simulink subsystem "Communication_Simulator"  (R2024a)
settings: Solver=VariableStepAuto  StartTime=0.0  StopTime=10.0  RelTol=1e-3
undefined symbols (not defined in the file): paramRFSatLink, QAM, rfSatSourceSamplesPerSymbol, rfSatSourceSampleTime
libraries: commrflib2 x24, dspsigops x12, commrfcorlib x8, commfilt2 x8, commdigbbndam3 x8, dspsolvers x8, simulink x8, commrandsrc3 x4, commsink2 x4, commdemoslib x4, impairlib x4, commsync2 x4
(part 2 of 3)

== system Communication_Simulator/TT&C Communication/Ground Segment/BER Calculation ==
  note: BER Results (with reset)
  note: Bits
  note: Errors
  note: BER
  BER Measurements : Display
  Constant : Constant  Value=paramRFSatLink.resetBER  SampleTime=rfSatSourceSampleTime * rfSatSourceSamplesPerSymbol
  Error Rate Calculation : commsink2/Error Rate Calculation  N=24  st_delay=0  cp_mode=Entire frame  subframe=[]  PMode=Port  WsName=ErrorVec  RsMode2=on  stop=off  numErr=200  maxBits=1e6
  Selector : Selector  InputPortWidth=3  IndexOptions=Index vector (dialog)  Indices=[1]  OutputSizes=1
  BER : Outport  VectorParamsAs1DForOutWhenUnconnected=off
  wires:
  [RF_downlink_Tx] -> Error Rate Calculation/1
  Selector/1 -> BER/1
  Constant/1 -> Error Rate Calculation/3
  Error Rate Calculation/1 -> BER Measurements/1, Selector/1
  [RF_downlink_Rx] -> Error Rate Calculation/2

== system Communication_Simulator/TT&C Communication/Ground Segment/BER Calculation1 ==
  note: BER Results (with reset)
  note: Bits
  note: Errors
  note: BER
  BER Measurements : Display
  Constant : Constant  Value=paramRFSatLink.resetBER  SampleTime=rfSatSourceSampleTime * rfSatSourceSamplesPerSymbol
  Error Rate Calculation : commsink2/Error Rate Calculation  N=24  st_delay=0  cp_mode=Entire frame  subframe=[]  PMode=Port  WsName=ErrorVec  RsMode2=on  stop=off  numErr=200  maxBits=1e6
  Selector : Selector  InputPortWidth=3  IndexOptions=Index vector (dialog)  Indices=[1]  OutputSizes=1
  BER : Outport  VectorParamsAs1DForOutWhenUnconnected=off
  wires:
  [RF_uplink_Tx] -> Error Rate Calculation/1
  Selector/1 -> BER/1
  Constant/1 -> Error Rate Calculation/3
  Error Rate Calculation/1 -> BER Measurements/1, Selector/1
  [RF_uplink_Rx] -> Error Rate Calculation/2

== system Communication_Simulator/TT&C Communication/Ground Segment/Close Plots ==

== system Communication_Simulator/TT&C Communication/Ground Segment/Close Plots1 ==

== system Communication_Simulator/TT&C Communication/Ground Segment/Close Plots10 ==

== system Communication_Simulator/TT&C Communication/Ground Segment/Close Plots11 ==

== system Communication_Simulator/TT&C Communication/Ground Segment/Close Plots12 ==

== system Communication_Simulator/TT&C Communication/Ground Segment/Close Plots13 ==

== system Communication_Simulator/TT&C Communication/Ground Segment/Close Plots14 ==

== system Communication_Simulator/TT&C Communication/Ground Segment/Close Plots15 ==

== system Communication_Simulator/TT&C Communication/Ground Segment/Close Plots2 ==

== system Communication_Simulator/TT&C Communication/Ground Segment/Close Plots3 ==

== system Communication_Simulator/TT&C Communication/Ground Segment/Close Plots4 ==

== system Communication_Simulator/TT&C Communication/Ground Segment/Close Plots5 ==

== system Communication_Simulator/TT&C Communication/Ground Segment/Close Plots6 ==

== system Communication_Simulator/TT&C Communication/Ground Segment/Close Plots7 ==

== system Communication_Simulator/TT&C Communication/Ground Segment/Close Plots8 ==

== system Communication_Simulator/TT&C Communication/Ground Segment/Close Plots9 ==

== system Communication_Simulator/TT&C Communication/Ground Segment/Downlink ==
  note: Downlink Path
  note: Satellite Downlink Transmitter
  note: Transmitter
  Telemetry : Inport
  Doppler Error : commrflib2/Phase// Frequency Offset  phaseOffset=0  freqPort=off  freqOffset=paramRFSatLink.DoppOffset
  Downlink Path : commrflib2/Free Space Path Loss  mode=Distance and Frequency  dB=180  d=paramRFSatLink.Altitude  fc=paramRFSatLink.Frequency
  Nonlinearity : Subsystem
      mask Display: disp('HPA\n Nonlinearity\n with Optional\n Digital\nPredistortion')
  Raised Cosine Transmit Filter : commfilt2/Raised Cosine Transmit Filter  filtType=Square root  R=0.3  filtSpan=paramRFSatLink.FilterSpan  N=paramRFSatLink.SamplesPerSymbol  filterGain=sqrt(paramRFSatLink.SamplesPerSymbol)  InputProcessing=Columns as channels (frame based)  RateOptions=Enforce single-rate processing  framing=Mute  checkCoeff=off  variableName=rcTxFilt  checkGain=Normalized  sampMode=Mute  saveAsFlag=0  currentFiltSpan=2*((2*(3))/2)  D=(2*(3))/2  launchFVT=off  roundingMode=Floor  overflowMode=off  coeffDataTypeStr=Inherit: Same word length as input  coeffMin=[]  coeffMax=[]  coeffLastDataTypeStr=Inherit: Same word length as input  outputDataTypeStr=Inherit: Same as accumulator  outputMin=[]  outputMax=[]  outputLastDataTypeStr=Inherit: Same as accumulator
  Rectangular QAM Modulator Baseband : commdigbbndam3/Rectangular QAM Modulator Baseband  M=16  InType=Bit  Enc=Gray  Mapping=[0:15]  PowType=Average Power  MinDist=2  AvgPow=2  PeakPow=1  Ph=0  outDtype=double  outWordLen=16  outUDDataType=sfix(16)  outFracLenMode=Best precision  outFracLen=15  outDataTypeStr=double  outLastDataTypeStr=double
  Tx Dish Antenna Gain : Gain  Gain=paramRFSatLink.TXAntGain_Downlink  SaturateOnIntegerOverflow=on  OutDataTypeStr=Inherit: Same as input  ParamDataTypeStr=Inherit: Same as input
  gs_rx_sig : Outport
  tag scope: RF_downlink_Tx=global, Tx_downlink_Ampl=global, Tx_downlink_RRC=global
  wires:
  Tx Dish Antenna Gain/1 -> Downlink Path/1
  Downlink Path/1 -> Doppler Error/1
  Doppler Error/1 -> gs_rx_sig/1
  Telemetry/1 -> [RF_downlink_Tx], Rectangular QAM Modulator Baseband/1
  Nonlinearity/1(Out2) -> Tx Dish Antenna Gain/1, [Tx_downlink_Ampl]
  Rectangular QAM Modulator Baseband/1 -> Raised Cosine Transmit Filter/1
  Raised Cosine Transmit Filter/1 -> Nonlinearity/1(In), [Tx_downlink_RRC]

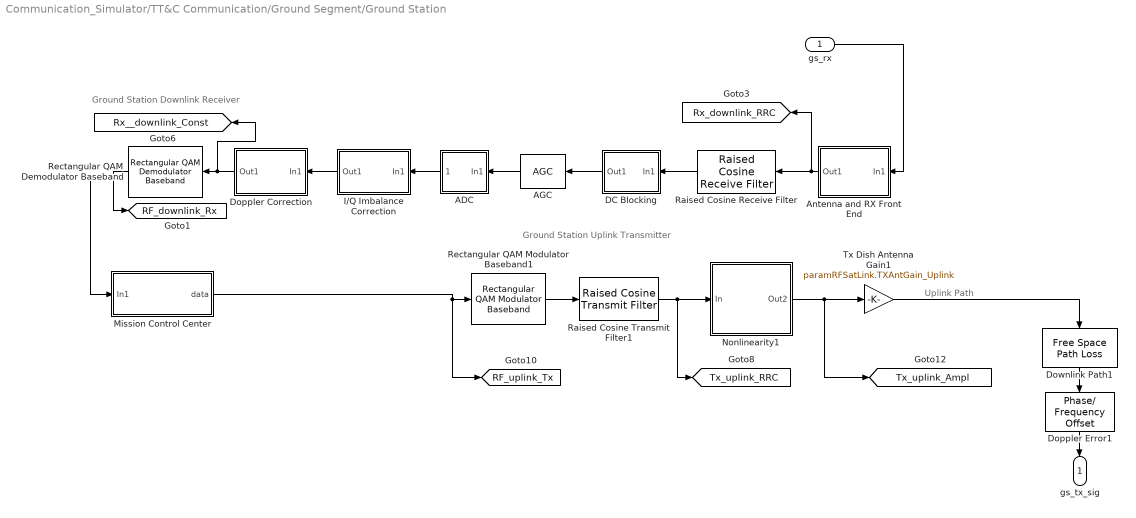
== system Communication_Simulator/TT&C Communication/Ground Segment/Ground Station ==
  note: Uplink Path
  note: Ground Station Uplink Transmitter
  note: Ground Station Downlink Receiver
  gs_rx : Inport
  ADC : Subsystem
      mask Display: disp('Bipolar\nADC')
  AGC : commrfcorlib/AGC  LegacyMode=off  DetectorMethod=Rectifier  LoopMethod=Linear  UpdatePeriod=100  StepSize=0.1  AdaptationStepSize=0.01  DesiredOutputPower=1  AveragingLength=256  MaximumGain=30  MaxPowerGain=400  GainOutputPort=off  InputPowerOutputPort=off  SimulateUsing=Code generation
  Antenna and RX Front End : Subsystem
      mask Display: disp('Antenna\nand\nRX Front End')
  DC Blocking : Subsystem
      mask Display: disp('DC\nBlocking')
  Doppler Correction : Subsystem
      mask Display: disp('Doppler\nCorrection')
  Doppler Error1 : commrflib2/Phase// Frequency Offset  phaseOffset=0  freqPort=off  freqOffset=paramRFSatLink.DoppOffset
  Downlink Path1 : commrflib2/Free Space Path Loss  mode=Distance and Frequency  dB=180  d=paramRFSatLink.Altitude  fc=paramRFSatLink.Frequency
  I/Q Imbalance Correction : Subsystem
      mask Display: disp('I/Q Imbalance\nCorrection')
  Mission Control Center : Subsystem
  Nonlinearity1 : Subsystem
      mask Display: disp('HPA\n Nonlinearity\n with Optional\n Digital\nPredistortion')
  Raised Cosine Receive Filter : commfilt2/Raised Cosine Receive Filter  filtType=Square root  R=0.3  filtSpan=paramRFSatLink.FilterSpan  N=paramRFSatLink.SamplesPerSymbol  downFactor=paramRFSatLink.SamplesPerSymbol  downOffset=0  filterGain=1/sqrt(paramRFSatLink.SamplesPerSymbol)  InputProcessing=Columns as channels (frame based)  RateOptions=Enforce single-rate processing  framing=Mute  checkCoeff=off  variableName=rcRxFilt  currentFiltSpan=2*((2*(3))/2)  D=(2*(3))/2  inputOffset=0  sampMode=Mute  saveAsFlag=0  rateMode=Downsampling  checkGain=Normalized  launchFVT=off  roundingMode=Floor  overflowMode=off  coeffDataTypeStr=Inherit: Same word length as input  coeffMin=[]  coeffMax=[]  coeffLastDataTypeStr=Inherit: Same word length as input  accumDataTypeStr=Inherit: Same as product output  accumLastDataTypeStr=Inherit: Same as product output  outputDataTypeStr=Inherit: Same as accumulator  outputMin=[]  outputMax=[]  outputLastDataTypeStr=Inherit: Same as accumulator
  Raised Cosine Transmit Filter1 : commfilt2/Raised Cosine Transmit Filter  filtType=Square root  R=0.3  filtSpan=paramRFSatLink.FilterSpan  N=paramRFSatLink.SamplesPerSymbol  filterGain=sqrt(paramRFSatLink.SamplesPerSymbol)  InputProcessing=Columns as channels (frame based)  RateOptions=Enforce single-rate processing  framing=Mute  checkCoeff=off  variableName=rcTxFilt1  checkGain=Normalized  sampMode=Mute  saveAsFlag=0  currentFiltSpan=2*((2*(3))/2)  D=(2*(3))/2  launchFVT=off  roundingMode=Floor  overflowMode=off  coeffDataTypeStr=Inherit: Same word length as input  coeffMin=[]  coeffMax=[]  coeffLastDataTypeStr=Inherit: Same word length as input  outputDataTypeStr=Inherit: Same as accumulator  outputMin=[]  outputMax=[]  outputLastDataTypeStr=Inherit: Same as accumulator
  Rectangular QAM Demodulator Baseband : commdigbbndam3/Rectangular QAM Demodulator Baseband  M=16  OutType=Bit  DecType=Hard decision  VarSource=Dialog  Variance=1  Dec=Gray  Mapping=[0:15]  PowType=Average Power  MinDist=2  AvgPow=2  PeakPow=1  Ph=0  outDtype1=double  outDtype2=double  derotateFactorWordLen=16  derotateFactorDataTypeStr=Inherit: Same word length as input  derotateFactorLastDataTypeStr=Inherit: Same word length as input  denormFactorWordLen=16  denormFactorDataTypeStr=Inherit: Same word length as input  denormFactorLastDataTypeStr=Inherit: Same word length as input  prodOutWordLen=32  prodOutOverflowMode=Wrap  prodOutRoundingMode=Floor  prodOutOvFlMode=off  prodOutOvFlModeLastStrValue=off  sumWordLen=32
  Rectangular QAM Modulator Baseband1 : commdigbbndam3/Rectangular QAM Modulator Baseband  M=16  InType=Bit  Enc=Gray  Mapping=[0:15]  PowType=Average Power  MinDist=2  AvgPow=1  PeakPow=1  Ph=0  outDtype=double  outWordLen=16  outUDDataType=sfix(16)  outFracLenMode=Best precision  outFracLen=15  outDataTypeStr=double  outLastDataTypeStr=double
  Tx Dish Antenna Gain1 : Gain  Gain=paramRFSatLink.TXAntGain_Uplink  SaturateOnIntegerOverflow=on  OutDataTypeStr=Inherit: Same as input  ParamDataTypeStr=Inherit: Same as input
  gs_tx_sig : Outport
  tag scope: RF_downlink_Rx=global, RF_uplink_Tx=global, Rx__downlink_Const=global, Rx_downlink_RRC=global, Tx_uplink_Ampl=global, Tx_uplink_RRC=global
  wires:
  Doppler Error1/1 -> gs_tx_sig/1
  Downlink Path1/1 -> Doppler Error1/1
  Tx Dish Antenna Gain1/1 -> Downlink Path1/1
  Rectangular QAM Modulator Baseband1/1 -> Raised Cosine Transmit Filter1/1
  Nonlinearity1/1(Out2) -> Tx Dish Antenna Gain1/1, [Tx_uplink_Ampl]
  Raised Cosine Transmit Filter1/1 -> Nonlinearity1/1(In), [Tx_uplink_RRC]
  Mission Control Center/1(data) -> [RF_uplink_Tx], Rectangular QAM Modulator Baseband1/1
  I/Q Imbalance Correction/1(Out1) -> Doppler Correction/1(In1)
  Antenna and RX Front End/1(Out1) -> [Rx_downlink_RRC], Raised Cosine Receive Filter/1
  DC Blocking/1(Out1) -> AGC/1
  ADC/1(Out2) -> I/Q Imbalance Correction/1(In1)
  Doppler Correction/1(Out1) -> Rectangular QAM Demodulator Baseband/1, [Rx__downlink_Const]
  AGC/1 -> ADC/1(In1)
  gs_rx/1 -> Antenna and RX Front End/1(In1)
  Raised Cosine Receive Filter/1 -> DC Blocking/1(In1)
  Rectangular QAM Demodulator Baseband/1 -> [RF_downlink_Rx], Mission Control Center/1(In1)

== system Communication_Simulator/TT&C Communication/Ground Segment/HPA ==
  HPA Input : Inport
  HPA Output : Inport  Port=2
  Matrix Concatenate : Concatenate  Mode=Multidimensional array  ConcatenateDimension=2
  RRC signal before and after HPA : ConstellationDiagram  WindowPosition=[508.333333333333 347.666666666667 282 242.666666666667]  SamplesPerSymbol=8  SymbolsToDisplaySource=Property  SymbolsToDisplay=1000  ReferenceConstellation=16-QAM  Title=RRC Signal Before and After HPA  XLimits=[-3.9233 3.9259]  YLimits=[-3.9233 3.9259]  ShowLegend=on  ShowReferenceConstellation=off  ColorFading=on  DefaultConfigurationName=comm.scopes.ConstellationDiagramBlockCfg
      settings: OpenAtSimulationStart=off
  wires:
  Matrix Concatenate/1 -> RRC signal before and after HPA/1
  HPA Output/1 -> Matrix Concatenate/2
  HPA Input/1 -> Matrix Concatenate/1

== system Communication_Simulator/TT&C Communication/Ground Segment/HPA1 ==
  HPA Input : Inport
  HPA Output : Inport  Port=2
  Matrix Concatenate : Concatenate  Mode=Multidimensional array  ConcatenateDimension=2
  RRC signal before and after HPA : ConstellationDiagram  WindowPosition=[508.333333333333 347.666666666667 282 242.666666666667]  SamplesPerSymbol=8  SymbolsToDisplaySource=Property  SymbolsToDisplay=1000  ReferenceConstellation=16-QAM  Title=RRC Signal Before and After HPA  XLimits=[-3.9233 3.9259]  YLimits=[-3.9233 3.9259]  ShowLegend=on  ShowReferenceConstellation=off  ColorFading=on  DefaultConfigurationName=comm.scopes.ConstellationDiagramBlockCfg
      settings: OpenAtSimulationStart=off
  wires:
  Matrix Concatenate/1 -> RRC signal before and after HPA/1
  HPA Output/1 -> Matrix Concatenate/2
  HPA Input/1 -> Matrix Concatenate/1

== system Communication_Simulator/TT&C Communication/Ground Segment/Input&Output of HPA ==
  In1 : Inport
  In2 : Inport  Port=2
  Add : Sum  Inputs=-+
  Complex to Magnitude-Angle : ComplexToMagnitudeAngle
  Complex to Magnitude-Angle1 : ComplexToMagnitudeAngle
  HPA AM to AM : ConstellationDiagram  Tag=ScatterPlot  WindowPosition=[1104 604 253 220]  SymbolsToDisplaySource=Property  SymbolsToDisplay=1000  Title=HPA AM to AM  XLimits=[-1.4713 6.1709]  YLimits=[-1.4713 6.1709]  XLabel=Input Amplitude  YLabel=Output Amplitude  ShowReferenceConstellation=off  ColorFading=on  DefaultConfigurationName=comm.scopes.ConstellationDiagramBlockCfg
      settings: OpenAtSimulationStart=off
  HPA AM to PM : ConstellationDiagram  Tag=ScatterPlot  WindowPosition=[842 605 253 220]  SymbolsToDisplaySource=Property  SymbolsToDisplay=1000  Title=HPA AM to PM  XLimits=[-1.0435 2.3201]  YLimits=[-1.0435 2.3201]  XLabel=Input Amplitude  YLabel=Phase Difference (rad)  ShowReferenceConstellation=off  ColorFading=on  DefaultConfigurationName=comm.scopes.ConstellationDiagramBlockCfg
      settings: OpenAtSimulationStart=off
  Real-Imag to Complex : RealImagToComplex
  Real-Imag to Complex1 : RealImagToComplex
  Unwrap : dspsigops/Unwrap  tol=pi  InputProcessing=Columns as channels (frame based)  running=on
  wires:
  Complex to Magnitude-Angle/2 -> Add/1
  Complex to Magnitude-Angle/1 -> Real-Imag to Complex/1, Real-Imag to Complex1/1
  Complex to Magnitude-Angle1/2 -> Add/2
  Unwrap/1 -> Real-Imag to Complex1/2
  Real-Imag to Complex1/1 -> HPA AM to PM/1
  In2/1 -> Complex to Magnitude-Angle1/1
  In1/1 -> Complex to Magnitude-Angle/1
  Add/1 -> Unwrap/1
  Complex to Magnitude-Angle1/1 -> Real-Imag to Complex/2
  Real-Imag to Complex/1 -> HPA AM to AM/1

== system Communication_Simulator/TT&C Communication/Ground Segment/Input&Output of HPA1 ==
  In1 : Inport
  In2 : Inport  Port=2
  Add : Sum  Inputs=-+
  Complex to Magnitude-Angle : ComplexToMagnitudeAngle
  Complex to Magnitude-Angle1 : ComplexToMagnitudeAngle
  HPA AM to AM : ConstellationDiagram  Tag=ScatterPlot  WindowPosition=[1104 604 253 220]  SymbolsToDisplaySource=Property  SymbolsToDisplay=1000  Title=HPA AM to AM  XLimits=[-1.4713 6.1709]  YLimits=[-1.4713 6.1709]  XLabel=Input Amplitude  YLabel=Output Amplitude  ShowReferenceConstellation=off  ColorFading=on  DefaultConfigurationName=comm.scopes.ConstellationDiagramBlockCfg
      settings: OpenAtSimulationStart=off
  HPA AM to PM : ConstellationDiagram  Tag=ScatterPlot  WindowPosition=[842 605 253 220]  SymbolsToDisplaySource=Property  SymbolsToDisplay=1000  Title=HPA AM to PM  XLimits=[-1.0435 2.3201]  YLimits=[-1.0435 2.3201]  XLabel=Input Amplitude  YLabel=Phase Difference (rad)  ShowReferenceConstellation=off  ColorFading=on  DefaultConfigurationName=comm.scopes.ConstellationDiagramBlockCfg
      settings: OpenAtSimulationStart=off
  Real-Imag to Complex : RealImagToComplex
  Real-Imag to Complex1 : RealImagToComplex
  Unwrap : dspsigops/Unwrap  tol=pi  InputProcessing=Columns as channels (frame based)  running=on
  wires:
  Complex to Magnitude-Angle/2 -> Add/1
  Complex to Magnitude-Angle/1 -> Real-Imag to Complex/1, Real-Imag to Complex1/1
  Complex to Magnitude-Angle1/2 -> Add/2
  Unwrap/1 -> Real-Imag to Complex1/2
  Real-Imag to Complex1/1 -> HPA AM to PM/1
  In2/1 -> Complex to Magnitude-Angle1/1
  In1/1 -> Complex to Magnitude-Angle/1
  Add/1 -> Unwrap/1
  Complex to Magnitude-Angle1/1 -> Real-Imag to Complex/2
  Real-Imag to Complex/1 -> HPA AM to AM/1

== system Communication_Simulator/TT&C Communication/Ground Segment/Power Spectrum ==
  In1 : Inport
  In2 : Inport  Port=2
  Matrix Concatenation : Concatenate  Mode=Multidimensional array  ConcatenateDimension=2
  Tx and Rx Spectrum : SpectrumAnalyzer  WindowPosition=[1.000000,41.000000,1020.000000,357.000000,]  ScopeFrameLocation=window  Method=Welch  SampleRate=200000  Span=200000  StartFrequency=-100000  StopFrequency=100000  AveragingMethod=Running  YLimits=[-132.25324983,35.45221687]  ShowLegend=on  ChannelNames="[\"Tramsitted \",\"Received\"]"  SelectedToolstripTab=spectrumAnalyzerToolstrip.spectrumTab  AllowFFTLengthLessThanSamplesPerUpdate=on  DefaultConfigurationName=spbscopes.SpectrumAnalyzerBlockCfg  IsFrequencyInputMode=0  FrequencyVectorPort=0  FrequencyVectorFromPort=0  FrequencyInputRBWPort=0  FrequencyInputRBWFromPort=0
  wires:
  Matrix Concatenation/1 -> Tx and Rx Spectrum/1
  In2/1 -> Matrix Concatenation/2
  In1/1 -> Matrix Concatenation/1

== system Communication_Simulator/TT&C Communication/Ground Segment/Power Spectrum1 ==
  In1 : Inport
  In2 : Inport  Port=2
  Matrix Concatenation : Concatenate  Mode=Multidimensional array  ConcatenateDimension=2
  Tx and Rx Spectrum : SpectrumAnalyzer  WindowPosition=[25 331 480 288]  Method=Welch  SampleRate=200000  Span=200000  StartFrequency=-100000  StopFrequency=100000  AveragingMethod=Running  YLimits=[-90.208205220815884218,27.456041881558888917]  ShowLegend=on  ChannelNames="[\"Tramsitted \",\"Received\"]"  AllowFFTLengthLessThanSamplesPerUpdate=on  DefaultConfigurationName=spbscopes.SpectrumAnalyzerBlockCfg  IsFrequencyInputMode=0  FrequencyVectorPort=0  FrequencyVectorFromPort=0  FrequencyInputRBWPort=0  FrequencyInputRBWFromPort=0
      settings: OpenAtSimulationStart=off
  wires:
  Matrix Concatenation/1 -> Tx and Rx Spectrum/1
  In2/1 -> Matrix Concatenation/2
  In1/1 -> Matrix Concatenation/1

== system Communication_Simulator/TT&C Communication/Ground Segment/Subsystem ==

== system Communication_Simulator/TT&C Communication/Ground Segment/Subsystem1 ==

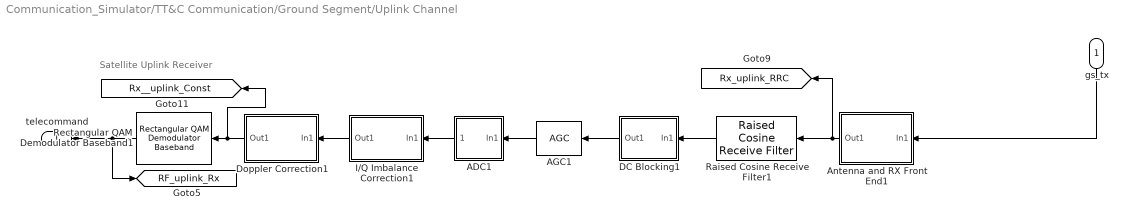
== system Communication_Simulator/TT&C Communication/Ground Segment/Uplink Channel ==
  note: Satellite Uplink Receiver
  gs_tx : Inport
  ADC1 : Subsystem
      mask Display: disp('Bipolar\nADC')
  AGC1 : commrfcorlib/AGC  LegacyMode=off  DetectorMethod=Rectifier  LoopMethod=Linear  UpdatePeriod=100  StepSize=0.1  AdaptationStepSize=0.01  DesiredOutputPower=1  AveragingLength=256  MaximumGain=30  MaxPowerGain=400  GainOutputPort=off  InputPowerOutputPort=off  SimulateUsing=Code generation
  Antenna and RX Front End1 : Subsystem
      mask Display: disp('Antenna\nand\nRX Front End')
  DC Blocking1 : Subsystem
      mask Display: disp('DC\nBlocking')
  Doppler Correction1 : Subsystem
      mask Display: disp('Doppler\nCorrection')
  I/Q Imbalance Correction1 : Subsystem
      mask Display: disp('I/Q Imbalance\nCorrection')
  Raised Cosine Receive Filter1 : commfilt2/Raised Cosine Receive Filter  filtType=Square root  R=0.3  filtSpan=paramRFSatLink.FilterSpan  N=paramRFSatLink.SamplesPerSymbol  downFactor=paramRFSatLink.SamplesPerSymbol  downOffset=0  filterGain=1/sqrt(paramRFSatLink.SamplesPerSymbol)  InputProcessing=Columns as channels (frame based)  RateOptions=Enforce single-rate processing  framing=Mute  checkCoeff=off  variableName=rcRxFilt1  currentFiltSpan=2*((2*(3))/2)  D=(2*(3))/2  inputOffset=0  sampMode=Mute  saveAsFlag=0  rateMode=Downsampling  checkGain=Normalized  launchFVT=off  roundingMode=Floor  overflowMode=off  coeffDataTypeStr=Inherit: Same word length as input  coeffMin=[]  coeffMax=[]  coeffLastDataTypeStr=Inherit: Same word length as input  accumDataTypeStr=Inherit: Same as product output  accumLastDataTypeStr=Inherit: Same as product output  outputDataTypeStr=Inherit: Same as accumulator  outputMin=[]  outputMax=[]  outputLastDataTypeStr=Inherit: Same as accumulator
  Rectangular QAM Demodulator Baseband1 : commdigbbndam3/Rectangular QAM Demodulator Baseband  M=16  OutType=Bit  DecType=Hard decision  VarSource=Dialog  Variance=1  Dec=Gray  Mapping=[0:15]  PowType=Average Power  MinDist=2  AvgPow=1  PeakPow=1  Ph=0  outDtype1=double  outDtype2=double  derotateFactorWordLen=16  derotateFactorDataTypeStr=Inherit: Same word length as input  derotateFactorLastDataTypeStr=Inherit: Same word length as input  denormFactorWordLen=16  denormFactorDataTypeStr=Inherit: Same word length as input  denormFactorLastDataTypeStr=Inherit: Same word length as input  prodOutWordLen=32  prodOutOverflowMode=Wrap  prodOutRoundingMode=Floor  prodOutOvFlMode=off  prodOutOvFlModeLastStrValue=off  sumWordLen=32
  telecommand : Outport
  tag scope: RF_uplink_Rx=global, Rx__uplink_Const=global, Rx_uplink_RRC=global
  wires:
  gs_tx/1 -> Antenna and RX Front End1/1(In1)
  I/Q Imbalance Correction1/1(Out1) -> Doppler Correction1/1(In1)
  Rectangular QAM Demodulator Baseband1/1 -> [RF_uplink_Rx], telecommand/1
  AGC1/1 -> ADC1/1(In1)
  Raised Cosine Receive Filter1/1 -> DC Blocking1/1(In1)
  ADC1/1(Out2) -> I/Q Imbalance Correction1/1(In1)
  Antenna and RX Front End1/1(Out1) -> [Rx_uplink_RRC], Raised Cosine Receive Filter1/1
  Doppler Correction1/1(Out1) -> Rectangular QAM Demodulator Baseband1/1, [Rx__uplink_Const]
  DC Blocking1/1(Out1) -> AGC1/1

== system Communication_Simulator/TT&C Communication/Ground Segment/background11 ==

== system Communication_Simulator/TT&C Communication/Ground Segment/background12 ==

== system Communication_Simulator/TT&C Communication/Ground Segment/background13 ==

== system Communication_Simulator/TT&C Communication/Ground Segment/background14 ==

== system Communication_Simulator/TT&C Communication/Ground Segment/background4 ==

== system Communication_Simulator/TT&C Communication/Ground Segment/background5 ==

== system Communication_Simulator/TT&C Communication/Ground Segment/background6 ==

== system Communication_Simulator/TT&C Communication/Ground Segment/background7 ==

== system Communication_Simulator/ISL Payload (SPARCS-B) /ISL/ISL Receiver/ADC1 ==
  In1 : Inport
  ADC Control : Constant  Value=paramRFSatLink.ADC  SampleTime=rfSatSourceSampleTime * rfSatSourceSamplesPerSymbol
  Bipolar ADC : commdemoslib/Bipolar ADC  FS_V=paramRFSatLink.ADC_VFS  N=paramRFSatLink.ADC_NumBits
  Switch : Switch  Criteria=u2 ~= 0  SaturateOnIntegerOverflow=off  InputSameDT=off
  Out2 : Outport  VectorParamsAs1DForOutWhenUnconnected=off
  wires:
  Switch/1 -> Out2/1
  In1/1 -> Switch/3, Bipolar ADC/1
  ADC Control/1 -> Switch/2
  Bipolar ADC/1 -> Switch/1

== system Communication_Simulator/ISL Payload (SPARCS-B) /ISL/ISL Receiver/Antenna and RX Front End1 ==
  In1 : Inport
  I/Q Imbalance : commrflib2/I//Q Imbalance  ampImbal=paramRFSatLink.IQImbal(1)  phsImbal=paramRFSatLink.IQImbal(2)  Idc=paramRFSatLink.IQImbal(3)  Qdc=paramRFSatLink.IQImbal(4)
  LNA : Gain  Gain=1e6
  Phase Noise : impairlib/Phase Noise  Level=rfSatPhaseNoise  FrequencyOffset=100  SampleRate=2e5  RandomStream=mt19937ar with seed  Seed=2137  SimulateUsing=Interpreted execution
  Rx Dish Antenna Gain : Gain  Gain=paramRFSatLink.RXAntGain_ISL  SaturateOnIntegerOverflow=on  OutDataTypeStr=Inherit: Same as input  ParamDataTypeStr=Inherit: Same as input
  Satellite Receiver System Temp : commrflib2/Receiver Thermal Noise  LegacyMode=on  NoiseMethod=Noise temperature  NoiseTemperature=paramRFSatLink.RXTemp  NoiseFigure=20  NoiseFactor=2  Add290KAntennaNoise=off  ReferenceLoad=1  RandomStream=mt19937ar with seed  Seed=67987  SimulateUsing=Code generation
  Out1 : Outport  VectorParamsAs1DForOutWhenUnconnected=off
  wires:
  Rx Dish Antenna Gain/1 -> Satellite Receiver System Temp/1
  I/Q Imbalance/1 -> LNA/1
  In1/1 -> Rx Dish Antenna Gain/1
  Satellite Receiver System Temp/1 -> Phase Noise/1
  Phase Noise/1 -> I/Q Imbalance/1
  LNA/1 -> Out1/1

== system Communication_Simulator/ISL Payload (SPARCS-B) /ISL/ISL Receiver/DC Blocking1 ==
  In1 : Inport
  DC Blocker : dspsigops/DC Blocker  Algorithm=IIR  NormalizedBandwidth=0.0005  Length=8  Order=3  SimulateUsing=Code generation
  DC Blocker Control : Constant  Value=paramRFSatLink.DCBlock  SampleTime=rfSatSourceSampleTime * rfSatSourceSamplesPerSymbol
  Switch : Switch  Criteria=u2 > Threshold  SaturateOnIntegerOverflow=off  InputSameDT=off
  Out1 : Outport  VectorParamsAs1DForOutWhenUnconnected=off
  wires:
  DC Blocker/1 -> Switch/1
  Switch/1 -> Out1/1
  DC Blocker Control/1 -> Switch/2
  In1/1 -> DC Blocker/1, Switch/3

== system Communication_Simulator/ISL Payload (SPARCS-B) /ISL/ISL Receiver/Doppler Correction1 ==
  In1 : Inport
  Carrier Synchronizer : commsync2/Carrier Synchronizer  Modulation=QAM  ModulationPhaseOffset=Auto  CustomPhaseOffset=0  SamplesPerSymbol=1  DampingFactor=0.707  NormalizedLoopBandwidth=0.001  EstimatedPhaseErrorOutputPort=off  SimulateUsing=Code generation
  Doppler Correction : Constant  Value=paramRFSatLink.CarrierSync  SampleTime=rfSatSourceSampleTime * rfSatSourceSamplesPerSymbol
  Switch : Switch  Criteria=u2 > Threshold  SaturateOnIntegerOverflow=off  InputSameDT=off
  Out1 : Outport  VectorParamsAs1DForOutWhenUnconnected=off
  wires:
  In1/1 -> Switch/3, Carrier Synchronizer/1
  Switch/1 -> Out1/1
  Carrier Synchronizer/1 -> Switch/1
  Doppler Correction/1 -> Switch/2

== system Communication_Simulator/ISL Payload (SPARCS-B) /ISL/ISL Receiver/I//Q Imbalance Correction1 ==
  In1 : Inport
  I/Q Imbalance Compensator : commrfcorlib/I//Q Imbalance Compensator  CoefficientSource=Estimated from input signal  InitialCoefficient=0 + 0j  StepSizeSource=Property  StepSize=0.00001  AdaptInputPort=off  CoefficientOutputPort=off  SimulateUsing=Code generation
  I/Q Imbalance Correction : Constant  Value=paramRFSatLink.IQComp  SampleTime=rfSatSourceSampleTime * rfSatSourceSamplesPerSymbol
  Switch : Switch  Criteria=u2 > Threshold  SaturateOnIntegerOverflow=off  InputSameDT=off
  Out1 : Outport  VectorParamsAs1DForOutWhenUnconnected=off
  wires:
  In1/1 -> Switch/3, I/Q Imbalance Compensator/1
  Switch/1 -> Out1/1
  I/Q Imbalance Compensator/1 -> Switch/1
  I/Q Imbalance Correction/1 -> Switch/2

== system Communication_Simulator/ISL Payload (SPARCS-B) /ISL/ISL Transmitter/Nonlinearity ==
  note: These two Memoryless Nonlinearity blocks should always
      | have the same settings.
  In : Inport
  Constant : Constant  Value=paramRFSatLink.preDistortion  VectorParams1D=off  SampleTime=rfSatSourceSampleTime * rfSatSourceSamplesPerSymbol
  Digital Pre-Distortion : Subsystem
      mask Display: disp('Digital\nPredistortion')
  Memoryless Nonlinearity : commrflib2/Memoryless Nonlinearity  Model=Saleh  LinearGainDB=0  TOI_Type=IIP3  IIP3=30  OIP3=Inf  IP1dB=Inf  OP1dB=Inf  IPsat=Inf  OPsat=Inf  Table=[ -25, 5, -1; -10, 20, -2; 0, 27, 5; 5, 28, 12 ]  MagnitudeGainDB=0  Vsat=1  MagnitudeSmooth=0.5  PhaseGainRadian=-.45  PhaseSaturation=.88  PhaseSmooth=3.43  InputScaleDB=paramRFSatLink.GindB  AmAmParameters=[2.1587 1.1517]  AmPmParameters=[4.0330 9.1040]  OutputScaleDB=paramRFSatLink.GoutdB  ReferenceLoad=1  SimulateUsing=Code generation
  Memoryless Nonlinearity1 : commrflib2/Memoryless Nonlinearity  Model=Saleh  LinearGainDB=0  TOI_Type=IIP3  IIP3=30  OIP3=Inf  IP1dB=Inf  OP1dB=Inf  IPsat=Inf  OPsat=Inf  Table=[ -25, 5, -1; -10, 20, -2; 0, 27, 5; 5, 28, 12 ]  MagnitudeGainDB=0  Vsat=1  MagnitudeSmooth=0.5  PhaseGainRadian=-.45  PhaseSaturation=.88  PhaseSmooth=3.43  InputScaleDB=paramRFSatLink.GindB  AmAmParameters=[2.1587 1.1517]  AmPmParameters=[4.0330 9.1040]  OutputScaleDB=paramRFSatLink.GoutdB  ReferenceLoad=1  SimulateUsing=Code generation
  Switch : Switch  Criteria=u2 > Threshold  Threshold=0.5  ZeroCross=off  SaturateOnIntegerOverflow=off  InputSameDT=off
  Out2 : Outport  VectorParamsAs1DForOutWhenUnconnected=off
  tag scope: HPA_In_isl=global, HPA_Out_isl=global
  wires:
  Memoryless Nonlinearity1/1 -> Switch/1
  Constant/1 -> Switch/2
  In/1 -> Digital Pre-Distortion/1(In1), Memoryless Nonlinearity/1, [HPA_In_isl]
  Switch/1 -> [HPA_Out_isl], Out2/1
  Memoryless Nonlinearity/1 -> Digital Pre-Distortion/2(In2), Switch/3
  Digital Pre-Distortion/1(Out1) -> Memoryless Nonlinearity1/1

== system Communication_Simulator/ISL Payload (SPARCS-B) /ISL/Other Satellite/ADC ==
  In1 : Inport
  ADC Control : Constant  Value=paramRFSatLink.ADC  SampleTime=rfSatSourceSampleTime * rfSatSourceSamplesPerSymbol
  Bipolar ADC : commdemoslib/Bipolar ADC  FS_V=paramRFSatLink.ADC_VFS  N=paramRFSatLink.ADC_NumBits
  Switch : Switch  Criteria=u2 ~= 0  SaturateOnIntegerOverflow=off  InputSameDT=off
  Out2 : Outport  VectorParamsAs1DForOutWhenUnconnected=off
  wires:
  Switch/1 -> Out2/1
  In1/1 -> Switch/3, Bipolar ADC/1
  ADC Control/1 -> Switch/2
  Bipolar ADC/1 -> Switch/1

== system Communication_Simulator/ISL Payload (SPARCS-B) /ISL/Other Satellite/Antenna and RX Front End ==
  In1 : Inport
  I/Q Imbalance : commrflib2/I//Q Imbalance  ampImbal=paramRFSatLink.IQImbal(1)  phsImbal=paramRFSatLink.IQImbal(2)  Idc=paramRFSatLink.IQImbal(3)  Qdc=paramRFSatLink.IQImbal(4)
  LNA : Gain  Gain=1e6
  Phase Noise : impairlib/Phase Noise  Level=rfSatPhaseNoise  FrequencyOffset=100  SampleRate=2e5  RandomStream=mt19937ar with seed  Seed=2137  SimulateUsing=Interpreted execution
  Rx Dish Antenna Gain : Gain  Gain=paramRFSatLink.RXAntGain_ISL  SaturateOnIntegerOverflow=on  OutDataTypeStr=Inherit: Same as input  ParamDataTypeStr=Inherit: Same as input
  Satellite Receiver System Temp : commrflib2/Receiver Thermal Noise  LegacyMode=on  NoiseMethod=Noise temperature  NoiseTemperature=paramRFSatLink.RXTemp  NoiseFigure=20  NoiseFactor=2  Add290KAntennaNoise=off  ReferenceLoad=1  RandomStream=mt19937ar with seed  Seed=67987  SimulateUsing=Code generation
  Out1 : Outport  VectorParamsAs1DForOutWhenUnconnected=off
  wires:
  Rx Dish Antenna Gain/1 -> Satellite Receiver System Temp/1
  I/Q Imbalance/1 -> LNA/1
  In1/1 -> Rx Dish Antenna Gain/1
  Satellite Receiver System Temp/1 -> Phase Noise/1
  Phase Noise/1 -> I/Q Imbalance/1
  LNA/1 -> Out1/1

== system Communication_Simulator/ISL Payload (SPARCS-B) /ISL/Other Satellite/DC Blocking ==
  In1 : Inport
  DC Blocker : dspsigops/DC Blocker  Algorithm=IIR  NormalizedBandwidth=0.0005  Length=8  Order=3  SimulateUsing=Code generation
  DC Blocker Control : Constant  Value=paramRFSatLink.DCBlock  SampleTime=rfSatSourceSampleTime * rfSatSourceSamplesPerSymbol
  Switch : Switch  Criteria=u2 > Threshold  SaturateOnIntegerOverflow=off  InputSameDT=off
  Out1 : Outport  VectorParamsAs1DForOutWhenUnconnected=off
  wires:
  DC Blocker/1 -> Switch/1
  Switch/1 -> Out1/1
  DC Blocker Control/1 -> Switch/2
  In1/1 -> DC Blocker/1, Switch/3

== system Communication_Simulator/ISL Payload (SPARCS-B) /ISL/Other Satellite/Doppler Correction ==
  In1 : Inport
  Carrier Synchronizer : commsync2/Carrier Synchronizer  Modulation=QAM  ModulationPhaseOffset=Auto  CustomPhaseOffset=0  SamplesPerSymbol=1  DampingFactor=0.707  NormalizedLoopBandwidth=0.001  EstimatedPhaseErrorOutputPort=off  SimulateUsing=Code generation
  Doppler Correction : Constant  Value=paramRFSatLink.CarrierSync  SampleTime=rfSatSourceSampleTime * rfSatSourceSamplesPerSymbol
  Switch : Switch  Criteria=u2 > Threshold  SaturateOnIntegerOverflow=off  InputSameDT=off
  Out1 : Outport  VectorParamsAs1DForOutWhenUnconnected=off
  wires:
  In1/1 -> Switch/3, Carrier Synchronizer/1
  Switch/1 -> Out1/1
  Carrier Synchronizer/1 -> Switch/1
  Doppler Correction/1 -> Switch/2

== system Communication_Simulator/ISL Payload (SPARCS-B) /ISL/Other Satellite/I//Q Imbalance Correction ==
  In1 : Inport
  I/Q Imbalance Compensator : commrfcorlib/I//Q Imbalance Compensator  CoefficientSource=Estimated from input signal  InitialCoefficient=0 + 0j  StepSizeSource=Property  StepSize=0.00001  AdaptInputPort=off  CoefficientOutputPort=off  SimulateUsing=Code generation
  I/Q Imbalance Correction : Constant  Value=paramRFSatLink.IQComp  SampleTime=rfSatSourceSampleTime * rfSatSourceSamplesPerSymbol
  Switch : Switch  Criteria=u2 > Threshold  SaturateOnIntegerOverflow=off  InputSameDT=off
  Out1 : Outport  VectorParamsAs1DForOutWhenUnconnected=off
  wires:
  In1/1 -> Switch/3, I/Q Imbalance Compensator/1
  Switch/1 -> Out1/1
  I/Q Imbalance Compensator/1 -> Switch/1
  I/Q Imbalance Correction/1 -> Switch/2

== system Communication_Simulator/ISL Payload (SPARCS-B) /ISL/Other Satellite/Nonlinearity1 ==
  note: These two Memoryless Nonlinearity blocks should always
      | have the same settings.
  In : Inport
  Constant : Constant  Value=paramRFSatLink.preDistortion  VectorParams1D=off  SampleTime=rfSatSourceSampleTime * rfSatSourceSamplesPerSymbol
  Digital Pre-Distortion : Subsystem
      mask Display: disp('Digital\nPredistortion')
  Memoryless Nonlinearity : commrflib2/Memoryless Nonlinearity  Model=Saleh  LinearGainDB=0  TOI_Type=IIP3  IIP3=30  OIP3=Inf  IP1dB=Inf  OP1dB=Inf  IPsat=Inf  OPsat=Inf  Table=[ -25, 5, -1; -10, 20, -2; 0, 27, 5; 5, 28, 12 ]  MagnitudeGainDB=0  Vsat=1  MagnitudeSmooth=0.5  PhaseGainRadian=-.45  PhaseSaturation=.88  PhaseSmooth=3.43  InputScaleDB=paramRFSatLink.GindB  AmAmParameters=[2.1587 1.1517]  AmPmParameters=[4.0330 9.1040]  OutputScaleDB=paramRFSatLink.GoutdB  ReferenceLoad=1  SimulateUsing=Code generation
  Memoryless Nonlinearity1 : commrflib2/Memoryless Nonlinearity  Model=Saleh  LinearGainDB=0  TOI_Type=IIP3  IIP3=30  OIP3=Inf  IP1dB=Inf  OP1dB=Inf  IPsat=Inf  OPsat=Inf  Table=[ -25, 5, -1; -10, 20, -2; 0, 27, 5; 5, 28, 12 ]  MagnitudeGainDB=0  Vsat=1  MagnitudeSmooth=0.5  PhaseGainRadian=-.45  PhaseSaturation=.88  PhaseSmooth=3.43  InputScaleDB=paramRFSatLink.GindB  AmAmParameters=[2.1587 1.1517]  AmPmParameters=[4.0330 9.1040]  OutputScaleDB=paramRFSatLink.GoutdB  ReferenceLoad=1  SimulateUsing=Code generation
  Switch : Switch  Criteria=u2 > Threshold  Threshold=0.5  ZeroCross=off  SaturateOnIntegerOverflow=off  InputSameDT=off
  Out2 : Outport  VectorParamsAs1DForOutWhenUnconnected=off
  tag scope: HPA_In_isl_Return=global, HPA_Out_isl_Return=global
  wires:
  Memoryless Nonlinearity1/1 -> Switch/1
  Constant/1 -> Switch/2
  In/1 -> Digital Pre-Distortion/1(In1), Memoryless Nonlinearity/1, [HPA_In_isl_Return]
  Switch/1 -> [HPA_Out_isl_Return], Out2/1
  Memoryless Nonlinearity/1 -> Digital Pre-Distortion/2(In2), Switch/3
  Digital Pre-Distortion/1(Out1) -> Memoryless Nonlinearity1/1

== system Communication_Simulator/ISL Payload (SPARCS-B) /ISL/Other Satellite/Other Satellite's OBC ==
  In1 : Inport
  Bernoulli Binary Generator : commrandsrc3/Bernoulli Binary Generator  ProbabilityOfZero=0.5  SeedSource=Parameter  Seed=37  SampleTime=rfSatSourceSampleTime  SamplesPerFrame=rfSatSourceSamplesPerSymbol  OutputDataType=double  SimulateUsing=Interpreted execution
  Terminator : Terminator
  data : Outport
  wires:
  Bernoulli Binary Generator/1 -> data/1
  In1/1 -> Terminator/1

== system Communication_Simulator/TT&C Communication/Ground Segment/Downlink/Nonlinearity ==
  note: These two Memoryless Nonlinearity blocks should always
      | have the same settings.
  In : Inport
  Constant : Constant  Value=paramRFSatLink.preDistortion  VectorParams1D=off  SampleTime=rfSatSourceSampleTime * rfSatSourceSamplesPerSymbol
  Digital Pre-Distortion : Subsystem
      mask Display: disp('Digital\nPredistortion')
  Memoryless Nonlinearity : commrflib2/Memoryless Nonlinearity  Model=Saleh  LinearGainDB=0  TOI_Type=IIP3  IIP3=30  OIP3=Inf  IP1dB=Inf  OP1dB=Inf  IPsat=Inf  OPsat=Inf  Table=[ -25, 5, -1; -10, 20, -2; 0, 27, 5; 5, 28, 12 ]  MagnitudeGainDB=0  Vsat=1  MagnitudeSmooth=0.5  PhaseGainRadian=-.45  PhaseSaturation=.88  PhaseSmooth=3.43  InputScaleDB=paramRFSatLink.GindB  AmAmParameters=[2.1587 1.1517]  AmPmParameters=[4.0330 9.1040]  OutputScaleDB=paramRFSatLink.GoutdB  ReferenceLoad=1  SimulateUsing=Code generation
  Memoryless Nonlinearity1 : commrflib2/Memoryless Nonlinearity  Model=Saleh  LinearGainDB=0  TOI_Type=IIP3  IIP3=30  OIP3=Inf  IP1dB=Inf  OP1dB=Inf  IPsat=Inf  OPsat=Inf  Table=[ -25, 5, -1; -10, 20, -2; 0, 27, 5; 5, 28, 12 ]  MagnitudeGainDB=0  Vsat=1  MagnitudeSmooth=0.5  PhaseGainRadian=-.45  PhaseSaturation=.88  PhaseSmooth=3.43  InputScaleDB=paramRFSatLink.GindB  AmAmParameters=[2.1587 1.1517]  AmPmParameters=[4.0330 9.1040]  OutputScaleDB=paramRFSatLink.GoutdB  ReferenceLoad=1  SimulateUsing=Code generation
  Switch : Switch  Criteria=u2 > Threshold  Threshold=0.5  ZeroCross=off  SaturateOnIntegerOverflow=off  InputSameDT=off
  Out2 : Outport  VectorParamsAs1DForOutWhenUnconnected=off
  tag scope: HPA_In_downlink=global, HPA_Out_downlink=global
  wires:
  Memoryless Nonlinearity1/1 -> Switch/1
  Constant/1 -> Switch/2
  In/1 -> Digital Pre-Distortion/1(In1), Memoryless Nonlinearity/1, [HPA_In_downlink]
  Switch/1 -> [HPA_Out_downlink], Out2/1
  Memoryless Nonlinearity/1 -> Digital Pre-Distortion/2(In2), Switch/3
  Digital Pre-Distortion/1(Out1) -> Memoryless Nonlinearity1/1

== system Communication_Simulator/TT&C Communication/Ground Segment/Ground Station/ADC ==
  In1 : Inport
  ADC Control : Constant  Value=paramRFSatLink.ADC  SampleTime=rfSatSourceSampleTime * rfSatSourceSamplesPerSymbol
  Bipolar ADC : commdemoslib/Bipolar ADC  FS_V=paramRFSatLink.ADC_VFS  N=paramRFSatLink.ADC_NumBits
  Switch : Switch  Criteria=u2 ~= 0  SaturateOnIntegerOverflow=off  InputSameDT=off
  Out2 : Outport  VectorParamsAs1DForOutWhenUnconnected=off
  wires:
  Switch/1 -> Out2/1
  In1/1 -> Switch/3, Bipolar ADC/1
  ADC Control/1 -> Switch/2
  Bipolar ADC/1 -> Switch/1

== system Communication_Simulator/TT&C Communication/Ground Segment/Ground Station/Antenna and RX Front End ==
  In1 : Inport
  I/Q Imbalance : commrflib2/I//Q Imbalance  ampImbal=paramRFSatLink.IQImbal(1)  phsImbal=paramRFSatLink.IQImbal(2)  Idc=paramRFSatLink.IQImbal(3)  Qdc=paramRFSatLink.IQImbal(4)
  LNA : Gain  Gain=1e6
  Phase Noise : impairlib/Phase Noise  Level=rfSatPhaseNoise  FrequencyOffset=100  SampleRate=2e5  RandomStream=mt19937ar with seed  Seed=2137  SimulateUsing=Interpreted execution
  Rx Dish Antenna Gain : Gain  Gain=paramRFSatLink.RXAntGain_Downlink  SaturateOnIntegerOverflow=on  OutDataTypeStr=Inherit: Same as input  ParamDataTypeStr=Inherit: Same as input
  Satellite Receiver System Temp : commrflib2/Receiver Thermal Noise  LegacyMode=on  NoiseMethod=Noise temperature  NoiseTemperature=paramRFSatLink.RXTemp  NoiseFigure=20  NoiseFactor=2  Add290KAntennaNoise=off  ReferenceLoad=1  RandomStream=mt19937ar with seed  Seed=67987  SimulateUsing=Code generation
  Out1 : Outport  VectorParamsAs1DForOutWhenUnconnected=off
  wires:
  Rx Dish Antenna Gain/1 -> Satellite Receiver System Temp/1
  I/Q Imbalance/1 -> LNA/1
  In1/1 -> Rx Dish Antenna Gain/1
  Satellite Receiver System Temp/1 -> Phase Noise/1
  Phase Noise/1 -> I/Q Imbalance/1
  LNA/1 -> Out1/1

== system Communication_Simulator/TT&C Communication/Ground Segment/Ground Station/DC Blocking ==
  In1 : Inport
  DC Blocker : dspsigops/DC Blocker  Algorithm=IIR  NormalizedBandwidth=0.0005  Length=8  Order=3  SimulateUsing=Code generation
  DC Blocker Control : Constant  Value=paramRFSatLink.DCBlock  SampleTime=rfSatSourceSampleTime * rfSatSourceSamplesPerSymbol
  Switch : Switch  Criteria=u2 > Threshold  SaturateOnIntegerOverflow=off  InputSameDT=off
  Out1 : Outport  VectorParamsAs1DForOutWhenUnconnected=off
  wires:
  DC Blocker/1 -> Switch/1
  Switch/1 -> Out1/1
  DC Blocker Control/1 -> Switch/2
  In1/1 -> DC Blocker/1, Switch/3

== system Communication_Simulator/TT&C Communication/Ground Segment/Ground Station/Doppler Correction ==
  In1 : Inport
  Carrier Synchronizer : commsync2/Carrier Synchronizer  Modulation=QAM  ModulationPhaseOffset=Auto  CustomPhaseOffset=0  SamplesPerSymbol=1  DampingFactor=0.707  NormalizedLoopBandwidth=0.001  EstimatedPhaseErrorOutputPort=off  SimulateUsing=Code generation
  Doppler Correction : Constant  Value=paramRFSatLink.CarrierSync  SampleTime=rfSatSourceSampleTime * rfSatSourceSamplesPerSymbol
  Switch : Switch  Criteria=u2 > Threshold  SaturateOnIntegerOverflow=off  InputSameDT=off
  Out1 : Outport  VectorParamsAs1DForOutWhenUnconnected=off
  wires:
  In1/1 -> Switch/3, Carrier Synchronizer/1
  Switch/1 -> Out1/1
  Carrier Synchronizer/1 -> Switch/1
  Doppler Correction/1 -> Switch/2

== system Communication_Simulator/TT&C Communication/Ground Segment/Ground Station/I//Q Imbalance Correction ==
  In1 : Inport
  I/Q Imbalance Compensator : commrfcorlib/I//Q Imbalance Compensator  CoefficientSource=Estimated from input signal  InitialCoefficient=0 + 0j  StepSizeSource=Property  StepSize=0.00001  AdaptInputPort=off  CoefficientOutputPort=off  SimulateUsing=Code generation
  I/Q Imbalance Correction : Constant  Value=paramRFSatLink.IQComp  SampleTime=rfSatSourceSampleTime * rfSatSourceSamplesPerSymbol
  Switch : Switch  Criteria=u2 > Threshold  SaturateOnIntegerOverflow=off  InputSameDT=off
  Out1 : Outport  VectorParamsAs1DForOutWhenUnconnected=off
  wires:
  In1/1 -> Switch/3, I/Q Imbalance Compensator/1
  Switch/1 -> Out1/1
  I/Q Imbalance Compensator/1 -> Switch/1
  I/Q Imbalance Correction/1 -> Switch/2

== system Communication_Simulator/TT&C Communication/Ground Segment/Ground Station/Mission Control Center ==
  In1 : Inport
  Bernoulli Binary Generator : commrandsrc3/Bernoulli Binary Generator  ProbabilityOfZero=0.5  SeedSource=Parameter  Seed=37  SampleTime=rfSatSourceSampleTime  SamplesPerFrame=rfSatSourceSamplesPerSymbol  OutputDataType=double  SimulateUsing=Interpreted execution
  Terminator : Terminator
  data : Outport
  wires:
  Bernoulli Binary Generator/1 -> data/1
  In1/1 -> Terminator/1

== system Communication_Simulator/TT&C Communication/Ground Segment/Ground Station/Nonlinearity1 ==
  note: These two Memoryless Nonlinearity blocks should always
      | have the same settings.
  In : Inport
  Constant : Constant  Value=paramRFSatLink.preDistortion  VectorParams1D=off  SampleTime=rfSatSourceSampleTime * rfSatSourceSamplesPerSymbol
  Digital Pre-Distortion : Subsystem
      mask Display: disp('Digital\nPredistortion')
  Memoryless Nonlinearity : commrflib2/Memoryless Nonlinearity  Model=Saleh  LinearGainDB=0  TOI_Type=IIP3  IIP3=30  OIP3=Inf  IP1dB=Inf  OP1dB=Inf  IPsat=Inf  OPsat=Inf  Table=[ -25, 5, -1; -10, 20, -2; 0, 27, 5; 5, 28, 12 ]  MagnitudeGainDB=0  Vsat=1  MagnitudeSmooth=0.5  PhaseGainRadian=-.45  PhaseSaturation=.88  PhaseSmooth=3.43  InputScaleDB=paramRFSatLink.GindB  AmAmParameters=[2.1587 1.1517]  AmPmParameters=[4.0330 9.1040]  OutputScaleDB=paramRFSatLink.GoutdB  ReferenceLoad=1  SimulateUsing=Code generation
  Memoryless Nonlinearity1 : commrflib2/Memoryless Nonlinearity  Model=Saleh  LinearGainDB=0  TOI_Type=IIP3  IIP3=30  OIP3=Inf  IP1dB=Inf  OP1dB=Inf  IPsat=Inf  OPsat=Inf  Table=[ -25, 5, -1; -10, 20, -2; 0, 27, 5; 5, 28, 12 ]  MagnitudeGainDB=0  Vsat=1  MagnitudeSmooth=0.5  PhaseGainRadian=-.45  PhaseSaturation=.88  PhaseSmooth=3.43  InputScaleDB=paramRFSatLink.GindB  AmAmParameters=[2.1587 1.1517]  AmPmParameters=[4.0330 9.1040]  OutputScaleDB=paramRFSatLink.GoutdB  ReferenceLoad=1  SimulateUsing=Code generation
  Switch : Switch  Criteria=u2 > Threshold  Threshold=0.5  ZeroCross=off  SaturateOnIntegerOverflow=off  InputSameDT=off
  Out2 : Outport  VectorParamsAs1DForOutWhenUnconnected=off
  tag scope: HPA_In_uplink=global, HPA_Out_uplink=global
  wires:
  Memoryless Nonlinearity1/1 -> Switch/1
  Constant/1 -> Switch/2
  In/1 -> Digital Pre-Distortion/1(In1), Memoryless Nonlinearity/1, [HPA_In_uplink]
  Switch/1 -> [HPA_Out_uplink], Out2/1
  Memoryless Nonlinearity/1 -> Digital Pre-Distortion/2(In2), Switch/3
  Digital Pre-Distortion/1(Out1) -> Memoryless Nonlinearity1/1

== system Communication_Simulator/TT&C Communication/Ground Segment/Uplink Channel/ADC1 ==
  In1 : Inport
  ADC Control : Constant  Value=paramRFSatLink.ADC  SampleTime=rfSatSourceSampleTime * rfSatSourceSamplesPerSymbol
  Bipolar ADC : commdemoslib/Bipolar ADC  FS_V=paramRFSatLink.ADC_VFS  N=paramRFSatLink.ADC_NumBits
  Switch : Switch  Criteria=u2 ~= 0  SaturateOnIntegerOverflow=off  InputSameDT=off
  Out2 : Outport  VectorParamsAs1DForOutWhenUnconnected=off
  wires:
  Switch/1 -> Out2/1
  In1/1 -> Switch/3, Bipolar ADC/1
  ADC Control/1 -> Switch/2
  Bipolar ADC/1 -> Switch/1

== system Communication_Simulator/TT&C Communication/Ground Segment/Uplink Channel/Antenna and RX Front End1 ==
  In1 : Inport
  I/Q Imbalance : commrflib2/I//Q Imbalance  ampImbal=paramRFSatLink.IQImbal(1)  phsImbal=paramRFSatLink.IQImbal(2)  Idc=paramRFSatLink.IQImbal(3)  Qdc=paramRFSatLink.IQImbal(4)
  LNA : Gain  Gain=1e6
  Phase Noise : impairlib/Phase Noise  Level=rfSatPhaseNoise  FrequencyOffset=100  SampleRate=2e5  RandomStream=mt19937ar with seed  Seed=2137  SimulateUsing=Interpreted execution
  Rx Dish Antenna Gain : Gain  Gain=paramRFSatLink.RXAntGain_Uplink  SaturateOnIntegerOverflow=on  OutDataTypeStr=Inherit: Same as input  ParamDataTypeStr=Inherit: Same as input
  Satellite Receiver System Temp : commrflib2/Receiver Thermal Noise  LegacyMode=on  NoiseMethod=Noise temperature  NoiseTemperature=paramRFSatLink.RXTemp  NoiseFigure=20  NoiseFactor=2  Add290KAntennaNoise=off  ReferenceLoad=1  RandomStream=mt19937ar with seed  Seed=67987  SimulateUsing=Code generation
  Out1 : Outport  VectorParamsAs1DForOutWhenUnconnected=off
  wires:
  Rx Dish Antenna Gain/1 -> Satellite Receiver System Temp/1
  I/Q Imbalance/1 -> LNA/1
  In1/1 -> Rx Dish Antenna Gain/1
  Satellite Receiver System Temp/1 -> Phase Noise/1
  Phase Noise/1 -> I/Q Imbalance/1
  LNA/1 -> Out1/1

== system Communication_Simulator/TT&C Communication/Ground Segment/Uplink Channel/DC Blocking1 ==
  In1 : Inport
  DC Blocker : dspsigops/DC Blocker  Algorithm=IIR  NormalizedBandwidth=0.0005  Length=8  Order=3  SimulateUsing=Code generation
  DC Blocker Control : Constant  Value=paramRFSatLink.DCBlock  SampleTime=rfSatSourceSampleTime * rfSatSourceSamplesPerSymbol
  Switch : Switch  Criteria=u2 > Threshold  SaturateOnIntegerOverflow=off  InputSameDT=off
  Out1 : Outport  VectorParamsAs1DForOutWhenUnconnected=off
  wires:
  DC Blocker/1 -> Switch/1
  Switch/1 -> Out1/1
  DC Blocker Control/1 -> Switch/2
  In1/1 -> DC Blocker/1, Switch/3

== system Communication_Simulator/TT&C Communication/Ground Segment/Uplink Channel/Doppler Correction1 ==
  In1 : Inport
  Carrier Synchronizer : commsync2/Carrier Synchronizer  Modulation=QAM  ModulationPhaseOffset=Auto  CustomPhaseOffset=0  SamplesPerSymbol=1  DampingFactor=0.707  NormalizedLoopBandwidth=0.001  EstimatedPhaseErrorOutputPort=off  SimulateUsing=Code generation
  Doppler Correction : Constant  Value=paramRFSatLink.CarrierSync  SampleTime=rfSatSourceSampleTime * rfSatSourceSamplesPerSymbol
  Switch : Switch  Criteria=u2 > Threshold  SaturateOnIntegerOverflow=off  InputSameDT=off
  Out1 : Outport  VectorParamsAs1DForOutWhenUnconnected=off
  wires:
  In1/1 -> Switch/3, Carrier Synchronizer/1
  Switch/1 -> Out1/1
  Carrier Synchronizer/1 -> Switch/1
  Doppler Correction/1 -> Switch/2

== system Communication_Simulator/TT&C Communication/Ground Segment/Uplink Channel/I//Q Imbalance Correction1 ==
  In1 : Inport
  I/Q Imbalance Compensator : commrfcorlib/I//Q Imbalance Compensator  CoefficientSource=Estimated from input signal  InitialCoefficient=0 + 0j  StepSizeSource=Property  StepSize=0.00001  AdaptInputPort=off  CoefficientOutputPort=off  SimulateUsing=Code generation
  I/Q Imbalance Correction : Constant  Value=paramRFSatLink.IQComp  SampleTime=rfSatSourceSampleTime * rfSatSourceSamplesPerSymbol
  Switch : Switch  Criteria=u2 > Threshold  SaturateOnIntegerOverflow=off  InputSameDT=off
  Out1 : Outport  VectorParamsAs1DForOutWhenUnconnected=off
  wires:
  In1/1 -> Switch/3, I/Q Imbalance Compensator/1
  Switch/1 -> Out1/1
  I/Q Imbalance Compensator/1 -> Switch/1
  I/Q Imbalance Correction/1 -> Switch/2

== system Communication_Simulator/ISL Payload (SPARCS-B) /ISL/ISL Transmitter/Nonlinearity/Digital Pre-Distortion ==
  In1 : Inport
  In2 : Inport  Port=2
  Distortion compensation : Subsystem
  Parameter Estimation : Subsystem
  Out1 : Outport  VectorParamsAs1DForOutWhenUnconnected=off
  wires:
  In1/1 -> Distortion compensation/3(In), Parameter Estimation/1(DUT Input)
  Parameter Estimation/1(c) -> Distortion compensation/1(c)
  Parameter Estimation/2(d) -> Distortion compensation/2(d)
  Distortion compensation/1(Pre-distorted Signal) -> Out1/1
  In2/1 -> Parameter Estimation/2(DUT Output)

== system Communication_Simulator/ISL Payload (SPARCS-B) /ISL/Other Satellite/Nonlinearity1/Digital Pre-Distortion ==
  In1 : Inport
  In2 : Inport  Port=2
  Distortion compensation : Subsystem
  Parameter Estimation : Subsystem
  Out1 : Outport  VectorParamsAs1DForOutWhenUnconnected=off
  wires:
  In1/1 -> Distortion compensation/3(In), Parameter Estimation/1(DUT Input)
  Parameter Estimation/1(c) -> Distortion compensation/1(c)
  Parameter Estimation/2(d) -> Distortion compensation/2(d)
  Distortion compensation/1(Pre-distorted Signal) -> Out1/1
  In2/1 -> Parameter Estimation/2(DUT Output)
